simulink model "lab2"  (R2018b)
settings: Solver=VariableStepAuto  StartTime=0.0  StopTime=0  RelTol=1e-3
values from neighbouring files (symbols this model uses):
  snr = SNR_dB(i)    [sim_code.m]    (also in sim_code2.m)
libraries: commrandsrc3 x1
settings Model: Creator=DSP_08  LastModifiedBy=DSP_08

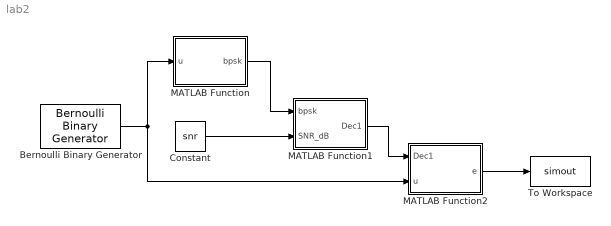
== system lab2 ==
  Bernoulli Binary Generator : commrandsrc3/Bernoulli Binary Generator  ProbabilityOfZero=0.5  SeedSource=Auto  Seed=0  SampleTime=1  SamplesPerFrame=100000  OutputDataType=double  SimulateUsing=Interpreted execution
  Constant : Constant  Value=snr
  MATLAB Function : MATLAB Function  TreatAsAtomicUnit=on
  MATLAB Function1 : MATLAB Function  TreatAsAtomicUnit=on
  MATLAB Function2 : MATLAB Function  TreatAsAtomicUnit=on
  To Workspace : ToWorkspace  VariableName=simout  SampleTime=-1
      settings: Save2DSignal=2-D array (concatenate along first dimension)
  wires:
  MATLAB Function/1(bpsk) -> MATLAB Function1/1(bpsk)
  MATLAB Function1/1(Dec1) -> MATLAB Function2/1(Dec1)
  MATLAB Function2/1(e) -> To Workspace/1
  Bernoulli Binary Generator/1 -> MATLAB Function2/2(u), MATLAB Function/1(u)
  Constant/1 -> MATLAB Function1/2(SNR_dB)

== matlab function lab2/MATLAB Function1 ==
  data: bpsk input; Dec1 output; SNR_dB input
function Dec1 = fcn(bpsk,SNR_dB)

    N = length(bpsk);
    h = complex(randn(1,N),randn(1,N));
    noise = complex(randn(1,N),randn(1,N));
    y = zeros(1,N) + 1j*zeros(1,N);
    Dec1 = zeros(1,N) + 1j*zeros(1,N);
    SNR_lin = 10^(SNR_dB/10);
    sigma = 1/sqrt(SNR_lin);
    
    y = h.*bpsk + sigma*noise;
    Dec1 = y./h;
    
end

== matlab function lab2/MATLAB Function ==
  data: u input; bpsk output
function bpsk = fcn(u)

    X = transpose(u);
    N = length(X);
    bpsk = zeros(1,N);
    for i = 1:N
        if X(i) == 0
            bpsk(i) = -1;
        else
            bpsk(i) = 1;
        end
    end
    
end

== matlab function lab2/MATLAB Function2 ==
  data: Dec1 input; e output; u input
function e = fcn(Dec1,u)

    N = length(Dec1);
    X = transpose(u);
    X_rcvd = zeros(1,N);
    
    for j = 1:N
        if Dec1(j) > 0
            X_rcvd(j) = 1;
        else
            X_rcvd(j) = 0;
        end
    end
    e = sum(abs(X-X_rcvd))/N;
    
end
